simulink model "sampleModel1681_5_sub_sub"  (R2023a)
settings: Solver=VariableStepAuto  StartTime=0.0  StopTime=10.0  RelTol=1e-3
libraries: hdlsllib x4, simulink x2
settings Model: Creator=user1  LastModifiedBy=user1

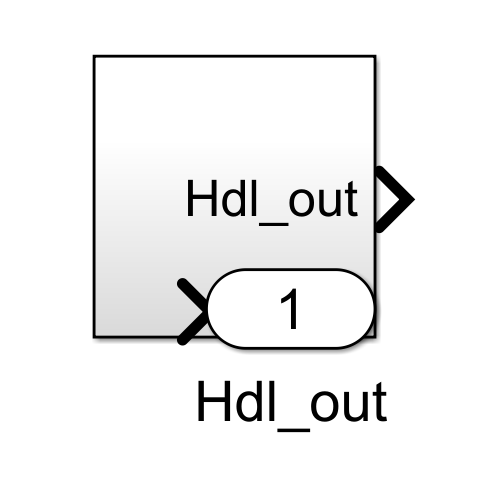
[thumbnail: Simulink's stored preview of the top-level diagram]
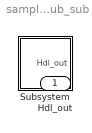
== system sampleModel1681_5_sub_sub ==
  Subsystem : Subsystem
  Hdl_out : Outport  OutDataTypeStr=uint8

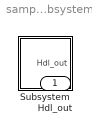
== system sampleModel1681_5_sub_sub/Subsystem ==
  Subsystem : Subsystem
  Hdl_out : Outport  OutDataTypeStr=uint8

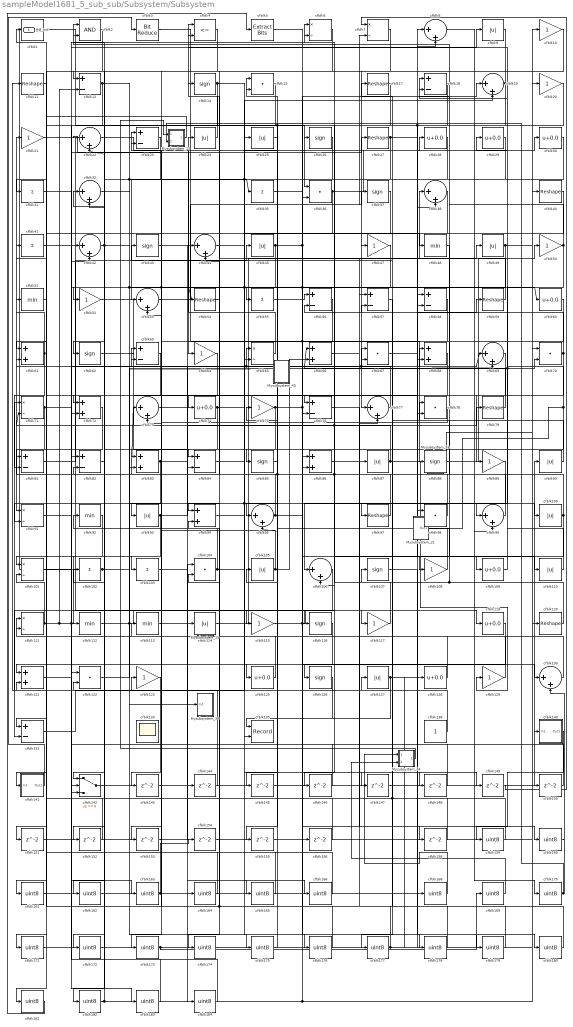
== system sampleModel1681_5_sub_sub/Subsystem/Subsystem ==
  Mysubsystem_13 : Subsystem  TreatAsAtomicUnit=on  RTWFcnName=Mysubsystem_13
      settings: RTWFcnNameOpts=User specified  RTWFileNameOpts=Use function name
  Mysubsystem_15 : Subsystem  TreatAsAtomicUnit=on  RTWFcnName=Mysubsystem_15
      settings: RTWFcnNameOpts=User specified  RTWFileNameOpts=Use function name
  Mysubsystem_21 : Subsystem  TreatAsAtomicUnit=on  RTWFcnName=Mysubsystem_21
      settings: RTWFcnNameOpts=User specified  RTWFileNameOpts=Use function name
  Mysubsystem_33 : Subsystem  TreatAsAtomicUnit=on  RTWFcnName=Mysubsystem_33
      settings: RTWFcnNameOpts=User specified  RTWFileNameOpts=Use function name
  Mysubsystem_34 : Subsystem  TreatAsAtomicUnit=on  RTWFcnName=Mysubsystem_34
      settings: RTWFcnNameOpts=User specified  RTWFileNameOpts=Use function name
  Mysubsystem_38 : Subsystem  TreatAsAtomicUnit=on  RTWFcnName=Mysubsystem_38
      settings: RTWFcnNameOpts=User specified  RTWFileNameOpts=Use function name
  Mysubsystem_43 : Subsystem  TreatAsAtomicUnit=on  RTWFcnName=Mysubsystem_43
      settings: RTWFcnNameOpts=User specified  RTWFileNameOpts=Use function name
  cfblk1 : simulink/Logic and Bit Operations/Bit Set  iBit=0
      settings: LibrarySourceBlock=|
      | hdlsllib/Logic and Bit
      | Operations/Bit Set
  cfblk{10,20..21,47,50,52,64,75,89,108,115,117,123,129} (14 alike) : Gain  OutDataTypeStr=uint8
  cfblk{9,24..25,45,49,87,90,93,100,105,110,114,127} (13 alike) : Abs  OutDataTypeStr=uint8  SaturateOnIntegerOverflow=off
  cfblk{6..7,65,71,91,101,111} (7 alike) : Product  Inputs=*/  OutDataTypeStr=uint8  RndMeth=Zero  SaturateOnIntegerOverflow=on
  cfblk{31,35,41,55,102..103} (6 alike) : Sum  Inputs=+  OutDataTypeStr=uint8
  cfblk{15,36,67,70,78,98,104,122} (8 alike) : DotProduct  OutDataTypeStr=uint8
  cfblk{8,19,22,32,38,42,44,53,69,73,77,95,99,106,130} (15 alike) : Sum  Inputs=|++  OutDataTypeStr=uint8
  cfblk{14,26,37,43,62,85,88,107,116,126} (10 alike) : Signum
  cfblk{28..30,60,74,109,119,125,128} (9 alike) : Bias  Bias=0.0  SaturateOnIntegerOverflow=off
  cfblk{11,17,27,40,54,59,79,97,120} (9 alike) : Reshape
  cfblk{48,51,92,112..113} (5 alike) : MinMax  OutDataTypeStr=uint8
  cfblk{12,18,23,56..58,63,76,81..82,84,131} (12 alike) : Sum  Inputs=+-  OutDataTypeStr=uint8
  cfblk{61,66,68,72,83,86,94,121} (8 alike) : Sum  OutDataTypeStr=uint8
  cfblk133 : Scope
      settings: Floating=on
  cfblk135 : Record  FileSettingsInternal="{\"entries\":[{\"content\":{\"excelSettings\":{\"content\":{},\"type\":\"Streamout.ExcelSettings\"}},\"type\":\"Streamout.FileSettingStorage\",\"uuid\":\"\"}],\"packageUris\":[\"http:\\/\\/schema.mathworks.com\\/mf0\\/streamout_blocks\\/R2020a\"],\"version\":\"1.0\"}"  Layout=[1 1]  SignalsInternal="{\"entries\":[{\"content\":{\"signals\":[{\"content\":{\"blockPath\":[],\"dimensions\":[1],\"domain\":\"\",\"lineColor\":\"#a2142f\",\"plots\":[1],\"port\":1,\"signalID\":34628,\"signalName\":\"cfblk126\"},\"type\":\"RecordBlkView.Signal\",\"uuid\":\"\"},{\"content\":{\"blockPath\":[],\"dimensions\":[1],\"domain\":\"\",\"lineColor\":\"#139fff\",\"plots\":[1],\"port\":2,\"signalID\":34631,\"signalName\":\"cfblk47\"},\"type\":\"RecordBlkView.Signal\",\"uuid\":\"\"}]},\"type\":\"RecordBlkView.InputSignals\",\"uuid\":\"\"}],\"packageUris\":[\"http:\\/\\/schema.mathworks.com\\/mf0\\/streamout_blocks\\/R2020a\"],\"version\":\"1.0\"}"  VisualizationBindings="{\"xyplotplugin\":{\"info\":[{\"series\":[{\"bindingParametersList\":[{\"parameter\":\"X-Axis\",\"signalID\":34628,\"signalName\":\"cfblk126\"},{\"parameter\":\"Y-Axis\",\"signalID\":34631,\"signalName\":\"cfblk47\"}],\"seriesID\":25063}],\"subplotID\":1}]}}"  CompatibilityTag=XY  st=-1
  cfblk138 : Constant  OutDataTypeStr=uint8  SampleTime=-1
  cfblk140 : Subsystem
      settings: LibrarySourceBlock=|
      | hdlsllib/Ports &
      | Subsystems/Subsystem
  cfblk141 : Subsystem
      settings: LibrarySourceBlock=|
      | hdlsllib/Ports &
      | Subsystems/Subsystem
  cfblk142 : Switch  OutDataTypeStr=uint8  SaturateOnIntegerOverflow=off  InputSameDT=off
  cfblk{143..156,158} (15 alike) : Delay  SampleTime=1
  cfblk{159..166,168..184} (25 alike) : DataTypeConversion  OutDataTypeStr=uint8  SaturateOnIntegerOverflow=off  RndMeth=Floor
  cfblk2 : Logic  AllPortsSameDT=off  OutDataTypeStr=boolean
  cfblk3 : hdlsllib/Logic and Bit Operations/Bit Reduce  mode=AND
  cfblk4 : RelationalOperator  Operator=<=  OutDataTypeStr=boolean  InputSameDT=off
  cfblk5 : simulink/Logic and Bit Operations/Extract Bits  bitsToExtract=Upper half  numBits=8  bitIdxRange=[0 7]  outScalingMode=Preserve fixed-point scaling
      settings: LibrarySourceBlock=|
      | hdlsllib/Logic and Bit
      | Operations/Extract Bits
  Hdl_out : Outport  OutDataTypeStr=uint8
  wires:
  Mysubsystem_34/1(Out1) -> Mysubsystem_13/1(In1)
  cfblk169/1 -> Mysubsystem_34/2(In2)
  cfblk168/1 -> Mysubsystem_34/1(In1)
  Mysubsystem_33/1(Out1) -> cfblk20/1
  Mysubsystem_21/1(Out1) -> cfblk4/2, cfblk172/1
  Mysubsystem_13/1(Out1) -> cfblk151/1
  cfblk184/1 -> cfblk82/2
  cfblk143/1 -> cfblk184/1
  cfblk183/1 -> cfblk82/1
  cfblk182/1 -> cfblk156/1, cfblk120/1, cfblk122/2
  cfblk181/1 -> cfblk5/1
  cfblk72/1 -> cfblk181/1
  cfblk180/1 -> cfblk121/2, cfblk104/2
  cfblk179/1 -> cfblk57/2
  cfblk178/1 -> cfblk57/1
  cfblk177/1 -> cfblk63/2, cfblk128/1
  cfblk176/1 -> cfblk102/1
  cfblk175/1 -> cfblk15/2
  cfblk102/1 -> cfblk175/1, Hdl_out/1
  cfblk174/1 -> cfblk10/1
  cfblk54/1 -> cfblk174/1
  cfblk173/1 -> cfblk169/1, cfblk150/1
  cfblk172/1 -> cfblk8/2
  cfblk171/1 -> cfblk8/1
  cfblk37/1 -> cfblk171/1
  cfblk170/1 -> Mysubsystem_13/2(In2), cfblk130/2
  cfblk107/1 -> cfblk168/1
  cfblk166/1 -> cfblk113/1
  cfblk165/1 -> cfblk123/1
  cfblk113/1 -> cfblk165/1
  cfblk164/1 -> cfblk41/1
  cfblk103/1 -> cfblk164/1
  cfblk163/1 -> cfblk154/1, cfblk38/2
  cfblk162/1 -> cfblk92/1
  cfblk161/1 -> cfblk86/1
  cfblk92/1 -> cfblk161/1
  cfblk160/1 -> cfblk140/1(In1)
  cfblk159/1 -> cfblk105/1, cfblk127/1
  cfblk158/1 -> cfblk17/1
  cfblk86/1 -> cfblk158/1
  cfblk156/1 -> cfblk1/1
  cfblk155/1 -> cfblk70/1
  cfblk154/1 -> cfblk36/2
  cfblk153/1 -> cfblk53/2
  cfblk152/1 -> cfblk111/2
  cfblk151/1 -> cfblk104/1
  cfblk150/1 -> cfblk122/1
  cfblk149/1 -> cfblk7/1
  cfblk35/1 -> cfblk149/1
  cfblk148/1 -> cfblk58/1
  cfblk44/1 -> cfblk148/1
  cfblk147/1 -> cfblk67/2
  cfblk146/1 -> cfblk23/2
  cfblk38/1 -> cfblk146/1
  cfblk145/1 -> cfblk77/2
  cfblk85/1 -> cfblk145/1
  cfblk144/1 -> cfblk71/1
  cfblk73/1 -> cfblk144/1
  cfblk123/1 -> cfblk143/1
  cfblk25/1 -> cfblk55/1
  cfblk60/1 -> cfblk76/2, cfblk83/1
  cfblk14/1 -> cfblk48/1, cfblk153/1
  cfblk117/1 -> cfblk71/2, cfblk63/1
  cfblk31/1 -> cfblk6/1
  cfblk48/1 -> cfblk108/1
  cfblk8/1 -> cfblk170/1
  cfblk49/1 -> cfblk40/1, cfblk72/2
  cfblk40/1 -> cfblk78/2
  cfblk19/1 -> cfblk76/1, cfblk12/1
  cfblk9/1 -> cfblk74/1
  cfblk120/1 -> cfblk61/2, cfblk98/2
  cfblk53/1 -> cfblk7/2
  cfblk32/1 -> Mysubsystem_38/1(In1), cfblk58/2
  cfblk91/1 -> cfblk42/2
  cfblk128/1 -> cfblk15/1
  cfblk94/1 -> cfblk28/1
  cfblk142/1 -> cfblk90/1
  cfblk79/1 -> cfblk18/1
  cfblk121/1 -> cfblk9/1, Mysubsystem_15/1(In1)
  cfblk90/1 -> cfblk43/1
  cfblk5/1 -> cfblk180/1
  cfblk74/1 -> cfblk19/2, cfblk152/1
  cfblk69/1 -> cfblk89/1
  cfblk130/1 -> cfblk107/1
  cfblk140/1(Out1) -> cfblk159/1
  cfblk62/1 -> cfblk98/1
  cfblk15/1 -> cfblk142/3
  cfblk101/1 -> cfblk42/1
  cfblk42/1 -> cfblk22/2, cfblk176/1
  cfblk76/1 -> cfblk87/1
  cfblk104/1 -> cfblk32/2, cfblk166/1
  cfblk50/1 -> cfblk2/1, cfblk99/1
  cfblk67/1 -> cfblk59/1
  cfblk56/1 -> cfblk95/1
  cfblk17/1 -> cfblk26/1
  cfblk82/1 -> cfblk182/1
  cfblk116/1 -> cfblk125/1
  cfblk112/1 -> cfblk115/1, cfblk69/2
  cfblk11/1 -> cfblk101/1
  cfblk110/1 -> cfblk66/1, cfblk18/2
  cfblk95/1 -> cfblk44/2, cfblk147/1
  cfblk28/1 -> cfblk85/1
  cfblk71/1 -> cfblk27/1, cfblk81/1
  cfblk129/1 -> cfblk94/2
  cfblk43/1 -> cfblk114/1
  cfblk30/1 -> cfblk116/1
  cfblk6/1 -> cfblk52/1
  cfblk122/1 -> cfblk70/2
  cfblk115/1 -> cfblk117/1, cfblk160/1
  cfblk68/1 -> cfblk126/1
  cfblk83/1 -> cfblk68/1, cfblk91/2
  cfblk27/1 -> cfblk53/1, cfblk110/1
  cfblk127/1 -> cfblk155/1, cfblk179/1
  cfblk18/1 -> cfblk61/1, cfblk95/2
  cfblk41/1 -> cfblk163/1
  cfblk89/1 -> cfblk106/1
  cfblk131/1 -> cfblk25/1
  cfblk45/1 -> cfblk83/2, cfblk103/1, cfblk60/1, cfblk130/1, cfblk37/1
  cfblk55/1 -> cfblk56/1
  cfblk23/1 -> cfblk72/1
  cfblk106/1 -> cfblk131/2
  cfblk12/1 -> cfblk100/1, cfblk54/1, cfblk35/1, cfblk142/2
  cfblk47/1 -> cfblk84/2, cfblk135/2
  cfblk58/1 -> cfblk97/1
  cfblk64/1 -> cfblk131/1
  cfblk109/1 -> cfblk29/1
  cfblk57/1 -> cfblk177/1
  cfblk108/1 -> cfblk23/1
  cfblk59/1 -> cfblk14/1
  cfblk105/1 -> cfblk73/2, cfblk66/2
  cfblk20/1 -> cfblk86/2, cfblk68/2
  cfblk66/1 -> cfblk49/1
  cfblk100/1 -> cfblk51/1, cfblk106/2
  cfblk126/1 -> cfblk135/1
  cfblk65/1 -> cfblk24/1
  cfblk75/1 -> cfblk109/1, cfblk19/1, cfblk94/1
  cfblk70/1 -> cfblk93/1, cfblk6/2
  cfblk111/1 -> cfblk69/1, cfblk65/1, cfblk183/1, cfblk12/2, cfblk101/2
  cfblk98/1 -> cfblk32/1, cfblk56/2
  cfblk10/1 -> cfblk173/1
  cfblk4/1 -> cfblk62/1
  cfblk84/1 -> cfblk99/2, cfblk178/1
  cfblk114/1 -> cfblk38/1
  cfblk99/1 -> cfblk78/1
  cfblk51/1 -> cfblk91/1
  cfblk1/1 -> cfblk36/1
  cfblk3/1 -> cfblk88/1
  cfblk29/1 -> cfblk47/1
  cfblk81/1 -> cfblk45/1
  cfblk141/1(Out1) -> cfblk3/1
  cfblk36/1 -> cfblk30/1, cfblk141/1(In1)
  cfblk97/1 -> cfblk73/1, cfblk75/1
  cfblk2/1 -> cfblk31/1
  cfblk26/1 -> cfblk65/2, cfblk162/1
  cfblk88/1 -> cfblk50/1
  cfblk22/1 -> cfblk64/1
  cfblk77/1 -> cfblk67/1, cfblk2/2
  cfblk61/1 -> cfblk21/1, cfblk81/2
  cfblk78/1 -> cfblk22/1
  cfblk7/1 -> cfblk77/1
  cfblk87/1 -> cfblk129/1, cfblk44/1
  cfblk119/1 -> cfblk121/1
  cfblk24/1 -> cfblk4/1
  cfblk63/1 -> cfblk142/1
  cfblk138/1 -> cfblk11/1
  cfblk125/1 -> cfblk111/1
  cfblk93/1 -> cfblk112/1, cfblk79/1
  cfblk52/1 -> cfblk84/1
  cfblk21/1 -> cfblk119/1

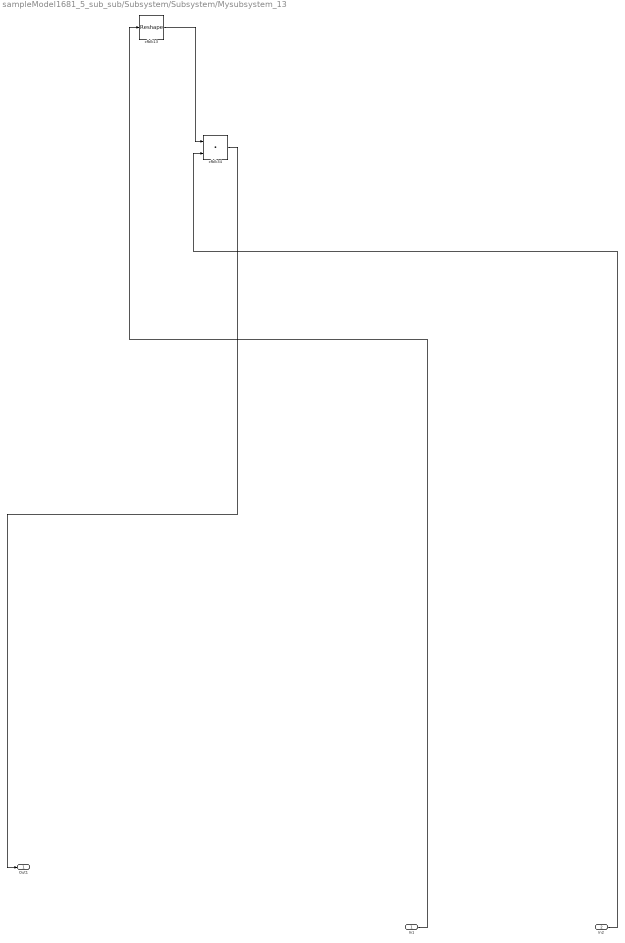
== system sampleModel1681_5_sub_sub/Subsystem/Subsystem/Mysubsystem_13 ==
  In1 : Inport
  In2 : Inport  Port=2
  cfblk13 : Reshape
  cfblk34 : DotProduct  OutDataTypeStr=Inherit: Inherit via internal rule
  Out1 : Outport
  wires:
  cfblk13/1 -> cfblk34/1
  In2/1 -> cfblk34/2
  In1/1 -> cfblk13/1
  cfblk34/1 -> Out1/1

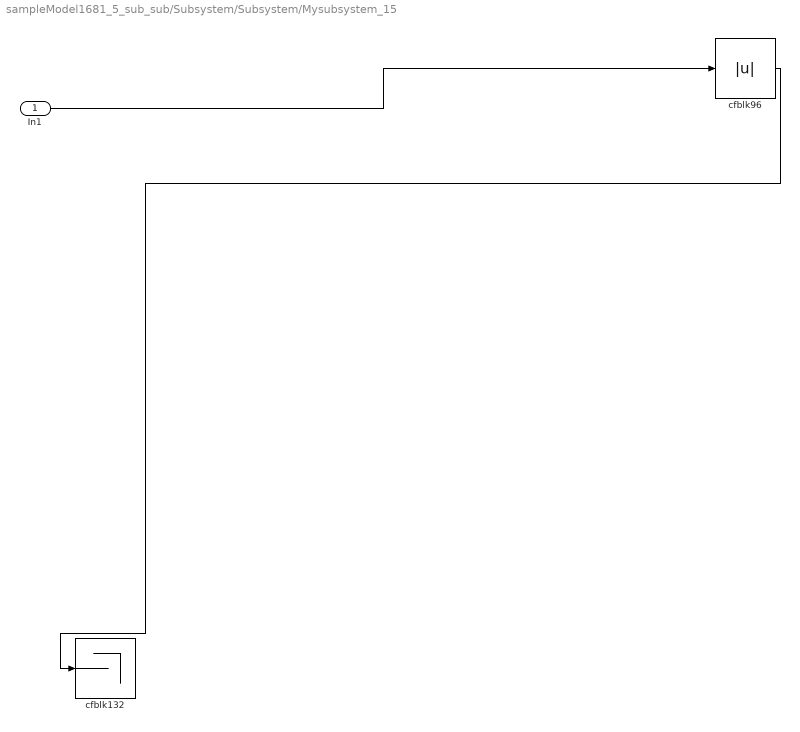
== system sampleModel1681_5_sub_sub/Subsystem/Subsystem/Mysubsystem_15 ==
  In1 : Inport
  cfblk132 : Terminator
  cfblk96 : Abs  SaturateOnIntegerOverflow=off
  wires:
  cfblk96/1 -> cfblk132/1
  In1/1 -> cfblk96/1

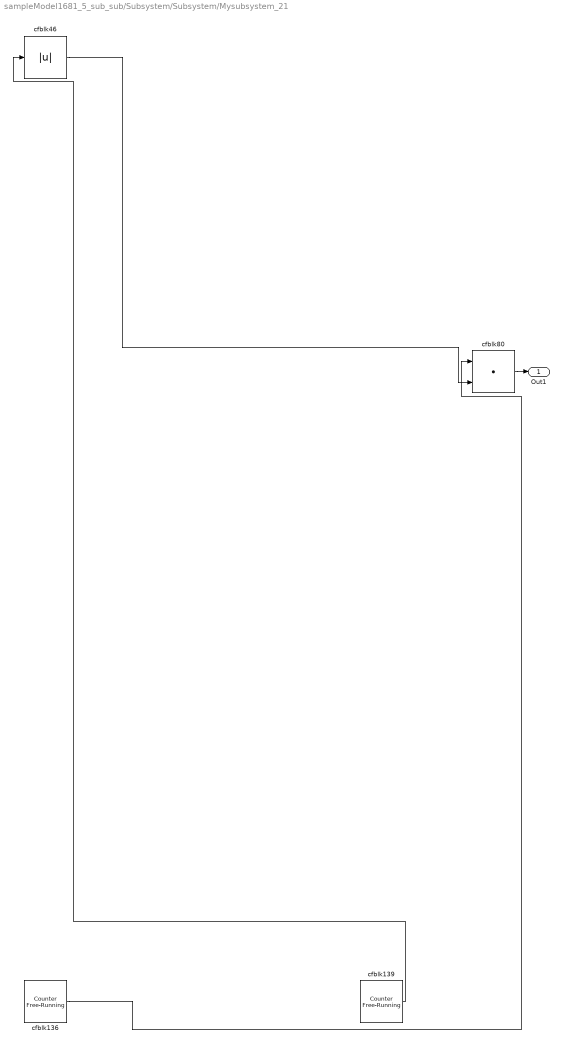
== system sampleModel1681_5_sub_sub/Subsystem/Subsystem/Mysubsystem_21 ==
  cfblk136 : hdlsllib/Sources/Counter Free-Running  NumBits=16  tsamp=-1
  cfblk139 : hdlsllib/Sources/Counter Free-Running  NumBits=16  tsamp=-1
  cfblk46 : Abs  SaturateOnIntegerOverflow=off
  cfblk80 : DotProduct  OutDataTypeStr=Inherit: Inherit via internal rule
  Out1 : Outport
  wires:
  cfblk46/1 -> cfblk80/2
  cfblk136/1 -> cfblk80/1
  cfblk139/1 -> cfblk46/1
  cfblk80/1 -> Out1/1

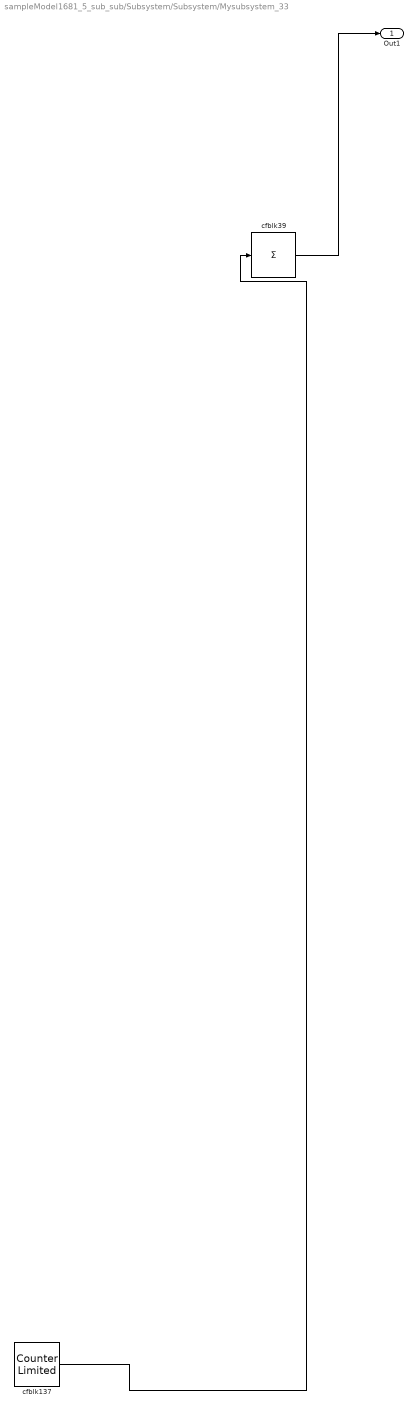
== system sampleModel1681_5_sub_sub/Subsystem/Subsystem/Mysubsystem_33 ==
  cfblk137 : hdlsllib/Sources/Counter Limited  uplimit=7  tsamp=-1
  cfblk39 : Sum  Inputs=+
  Out1 : Outport
  wires:
  cfblk137/1 -> cfblk39/1
  cfblk39/1 -> Out1/1

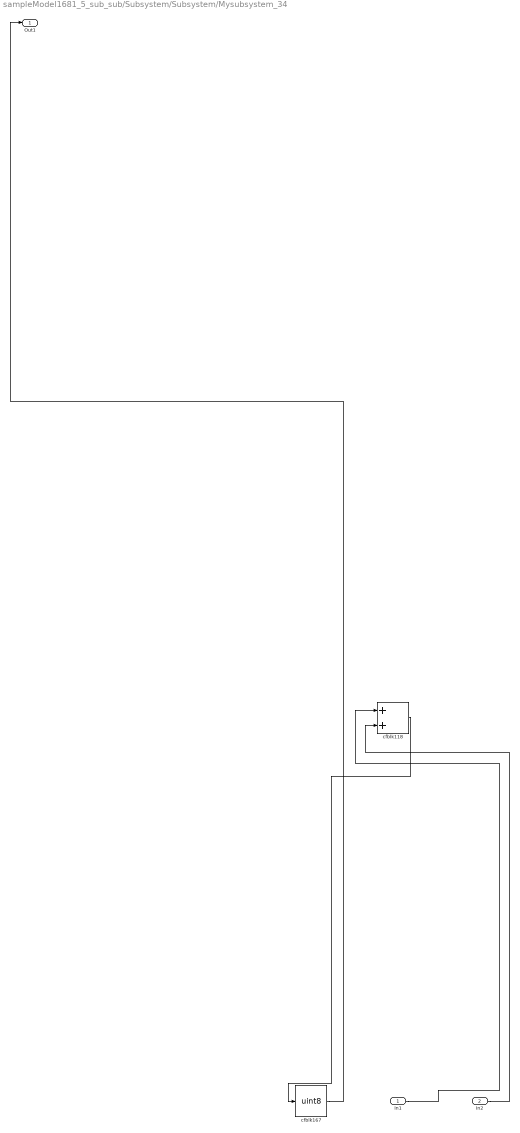
== system sampleModel1681_5_sub_sub/Subsystem/Subsystem/Mysubsystem_34 ==
  In1 : Inport
  In2 : Inport  Port=2
  cfblk118 : Sum
  cfblk167 : DataTypeConversion  OutDataTypeStr=uint8  SaturateOnIntegerOverflow=off  RndMeth=Floor
  Out1 : Outport
  wires:
  In2/1 -> cfblk118/2
  cfblk118/1 -> cfblk167/1
  In1/1 -> cfblk118/1
  cfblk167/1 -> Out1/1

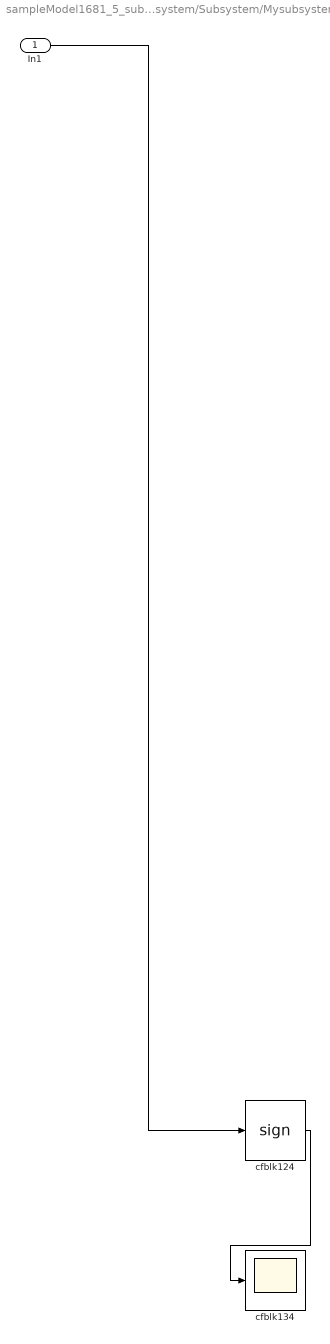
== system sampleModel1681_5_sub_sub/Subsystem/Subsystem/Mysubsystem_38 ==
  In1 : Inport
  cfblk124 : Signum
  cfblk134 : Scope
  wires:
  cfblk124/1 -> cfblk134/1
  In1/1 -> cfblk124/1

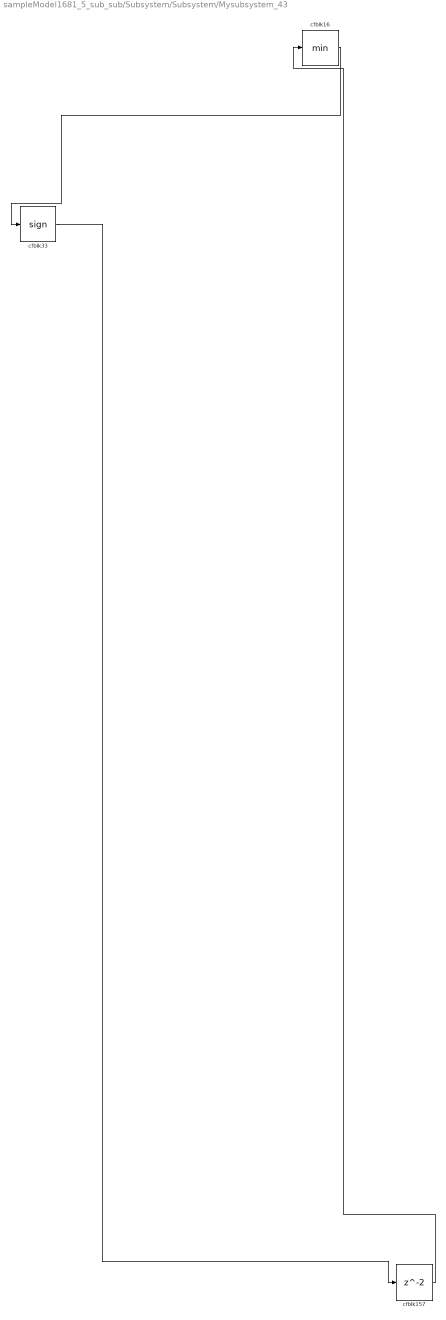
== system sampleModel1681_5_sub_sub/Subsystem/Subsystem/Mysubsystem_43 ==
  cfblk157 : Delay  SampleTime=1
  cfblk16 : MinMax
  cfblk33 : Signum
  wires:
  cfblk16/1 -> cfblk33/1
  cfblk33/1 -> cfblk157/1
  cfblk157/1 -> cfblk16/1

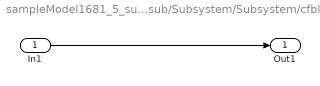
== system sampleModel1681_5_sub_sub/Subsystem/Subsystem/cfblk140 ==
  In1 : Inport
  Out1 : Outport
  wires:
  In1/1 -> Out1/1

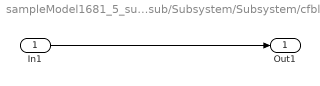
== system sampleModel1681_5_sub_sub/Subsystem/Subsystem/cfblk141 ==
  In1 : Inport
  Out1 : Outport
  wires:
  In1/1 -> Out1/1
